simulink library "fsw_out_bus"  (R2018b)
settings: Solver=VariableStepAuto  StartTime=0.0  StopTime=10.0  RelTol=1e-3
undefined symbols (not defined in the file): fswParams
settings Model: Creator=colem  LastModifiedBy=Nick's PC

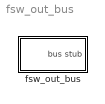
== system fsw_out_bus ==
  fsw_out_bus : Subsystem

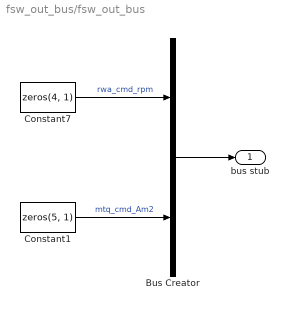
== system fsw_out_bus/fsw_out_bus ==
  Bus Creator : BusCreator  Inputs=2  OutDataTypeStr=Bus: fsw_out
  Constant1 : Constant  Value=zeros(5, 1)  SampleTime=fswParams.sample_time_s
  Constant7 : Constant  Value=zeros(4, 1)  SampleTime=fswParams.sample_time_s
  bus stub : Outport  OutDataTypeStr=Bus: fsw_out
  wires:
  Constant7/1 -> Bus Creator/1  "rwa_cmd_rpm"
  Bus Creator/1 -> bus stub/1
  Constant1/1 -> Bus Creator/2  "mtq_cmd_Am2"
